simulink model "simulink_test_controller"  (R2025b)
settings: Solver=FixedStepDiscrete  StartTime=0.0  StopTime=10.0  FixedStep=0.01  RelTol=1e-3
values from neighbouring files (symbols this model uses):
  workspace_matrix = workspace_scalar * eye(5)    [matlab_simulink_test_startup.m]    (also in precomputed.mat = [12340.5678 0 0 0 0 0 12340.5678 0 0 0 0 0 ... (25 elements,)
  workspace_scalar = 1234.5678    [matlab_simulink_test_startup.m]    (also in precomputed.mat = 12340.5678)
settings Model: Creator=leonardo-avoni  LastModifiedBy=leonardo-avoni

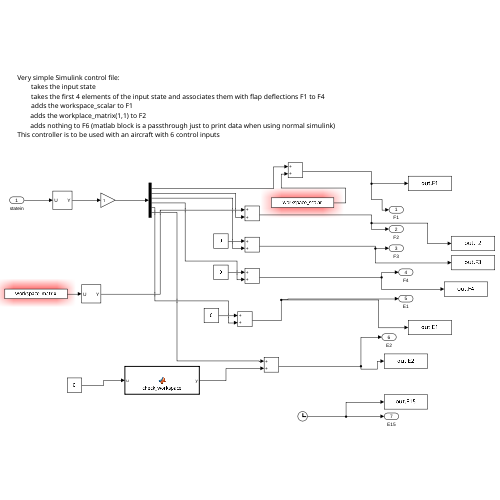
[thumbnail: Simulink's stored preview of the top-level diagram]
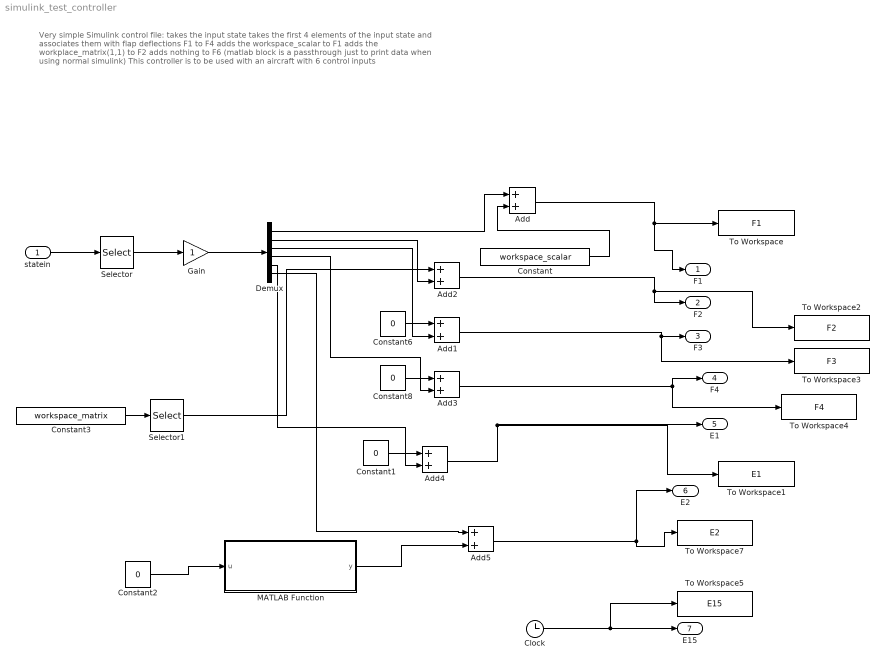
== system simulink_test_controller ==
  note: Very simple Simulink control file:
      | takes the input state
      | takes the first 4 elements of the input state and associates them with flap deflections F1 to F4
      | adds the workspace_scalar to F1
      | adds the workplace_matrix(1,1) to F2
      | adds nothing to F6 (matlab block is a passthrough just to print data when using normal simulink)
      | This controller is to be used with an aircraft with 6 control inputs
  statein : Inport  PortDimensions=1945
  Add{,1..5} (6 alike) : Sum
  Clock : Clock
  Constant : Constant  Value=workspace_scalar
  Constant{1..2,6,8} (4 alike) : Constant  Value=0
  Constant3 : Constant  Value=workspace_matrix
  Demux : Demux  Outputs=6
  Gain : Gain
  MATLAB Function : MATLAB Function  TreatAsAtomicUnit=on
  Selector : Selector  InputPortWidth=1945  IndexOptions=Index vector (dialog)  Indices=[1:6]  OutputSizes=1
  Selector1 : Selector  NumberOfDimensions=2  InputPortWidth=25  IndexOptions=Index vector (dialog),Index vector (dialog)  Indices=1,1  OutputSizes=1,1
  To Workspace : ToWorkspace  VariableName=F1  SaveFormat=Timeseries  SampleTime=-1
  To Workspace1 : ToWorkspace  VariableName=E1  SaveFormat=Timeseries  SampleTime=-1
  To Workspace2 : ToWorkspace  VariableName=F2  SaveFormat=Timeseries  SampleTime=-1
  To Workspace3 : ToWorkspace  VariableName=F3  SaveFormat=Timeseries  SampleTime=-1
  To Workspace4 : ToWorkspace  VariableName=F4  SaveFormat=Timeseries  SampleTime=-1
  To Workspace5 : ToWorkspace  VariableName=E15  SaveFormat=Timeseries  SampleTime=-1
  To Workspace7 : ToWorkspace  VariableName=E2  SaveFormat=Timeseries  SampleTime=-1
  F1 : Outport
  F2 : Outport  Port=2
  F3 : Outport  Port=3
  F4 : Outport  Port=4
  E1 : Outport  Port=5
  E2 : Outport  Port=6
  E15 : Outport  Port=7
  wires:
  Add/1 -> F1/1, To Workspace/1
  Add2/1 -> F2/1, To Workspace2/1
  Add1/1 -> To Workspace3/1, F3/1
  Add3/1 -> To Workspace4/1, F4/1
  statein/1 -> Selector/1
  Selector/1 -> Gain/1
  Gain/1 -> Demux/1
  Constant/1 -> Add/2
  Demux/1 -> Add/1
  Demux/2 -> Add2/2
  Selector1/1 -> Add2/1
  Constant8/1 -> Add3/1
  Demux/3 -> Add1/2
  Constant6/1 -> Add1/1
  Demux/4 -> Add3/2
  Constant1/1 -> Add4/1
  Add4/1 -> E1/1, To Workspace1/1
  Demux/5 -> Add4/2
  Demux/6 -> Add5/1
  Constant2/1 -> MATLAB Function/1(u)
  Constant3/1 -> Selector1/1
  MATLAB Function/1(y) -> Add5/2
  Add5/1 -> E2/1, To Workspace7/1
  Clock/1 -> E15/1, To Workspace5/1

== matlab function simulink_test_controller/MATLAB Function ==
  data: u input; y output
function y = check_workspace(u)

    coder.extrinsic('evalin');
    workspace_scalar = evalin('base','workspace_scalar');
    workspace_string  = evalin('base','workspace_string');
    workspace_matrix  = evalin('base','workspace_matrix');

    disp(workspace_scalar);
    disp(workspace_string);
    disp(workspace_matrix);
    y = u;  % Pass through input or compute
